simulink model "sampleModel137"  (R2021b)
settings: Solver=VariableStepAuto  StartTime=0.0  StopTime=10.0  RelTol=1e-3
undefined symbols (not defined in the file or in its folder): Newton, Raphson
libraries: simulink x11, slpidlib x2
settings Model: Creator=user  LastModifiedBy=user

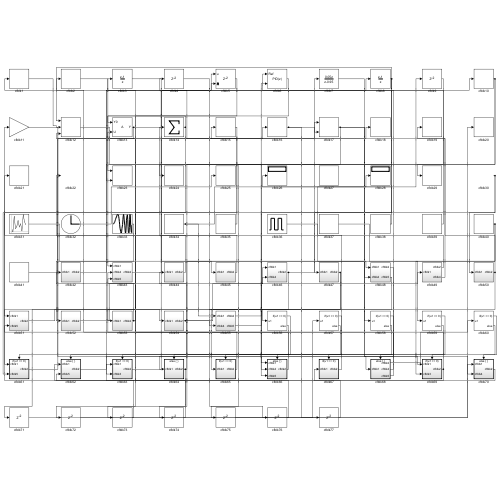
[thumbnail: Simulink's stored preview of the top-level diagram]
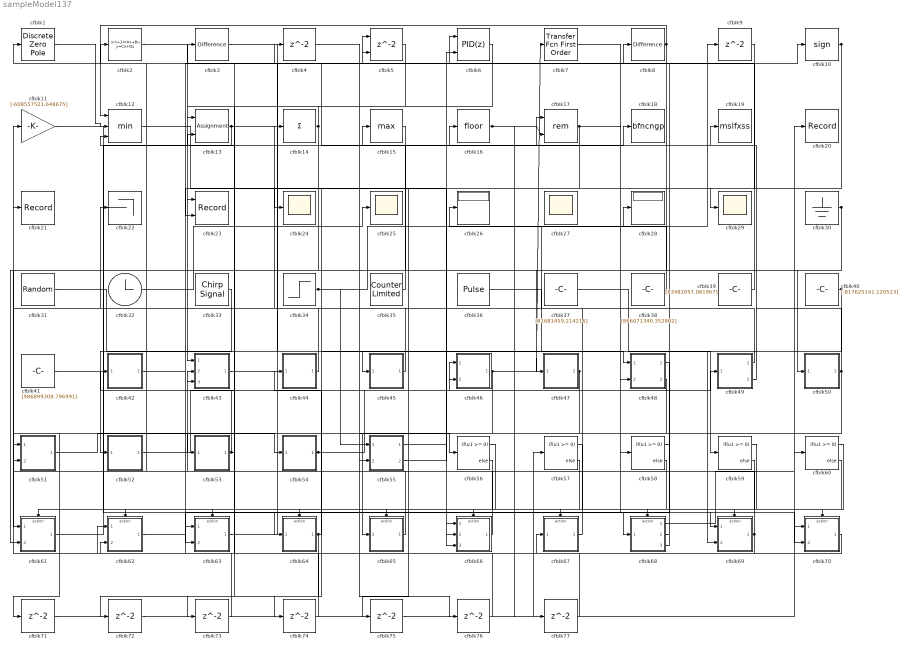
== system sampleModel137 ==
  cfblk1 : DiscreteZeroPole  Poles=[0 0.5]  Gain=1
  cfblk10 : Signum
  cfblk11 : Gain  Gain=[-608557521.648675]
  cfblk12 : MinMax  Inputs=3
  cfblk13 : Assignment  DiagnosticForDimensions=Warning  IndexOptions=Index vector (dialog)  Indices=1  OutputSizes=1
  cfblk14 : Sum  Inputs=+
  cfblk15 : MinMax  Function=max
  cfblk16 : Rounding
  cfblk17 : Math  Operator=rem  SaturateOnIntegerOverflow=on
  cfblk18 : ToWorkspace  VariableName=bfncngp  SaveFormat=Timeseries  SampleTime=-1
  cfblk19 : ToWorkspace  VariableName=mslfxss  SaveFormat=Timeseries  SampleTime=-1
  cfblk2 : DiscreteStateSpace
  cfblk20 : Record  FileSettingsInternal="{\"entries\":[{\"content\":{\"excelSettings\":{\"content\":{},\"type\":\"Streamout.ExcelSettings\"}},\"type\":\"Streamout.FileSettingStorage\",\"uuid\":\"78cab240-d707-46c0-bab2-71765f668cae\"}],\"packageUris\":[\"http://schema.mathworks.com/mf0/streamout_blocks/R2020a\"],\"version\":\"1.0\"}"  SignalsInternal="{\"entries\":[{\"content\":{\"signals\":[{\"content\":{\"blockPath\":[\"sampleModel137/cfblk20\"],\"channel\":[],\"dimensions\":[1],\"domain\":\"sampleModel137/cfblk20\",\"lineColor\":\"#77ac30\",\"plots\":[1],\"port\":1,\"sid\":[\"\"],\"signalID\":4817,\"signalName\":\"cfblk68:1\"},\"type\":\"RecordBlkView.Signal\",\"uuid\":\"5ba74064-0a93-45ca-96c5-9e64b5215f86\"}]},\"type\":\"RecordBlkView.InputSignals\",\"uuid\":\"459eb6df-0716-4f70-a343-e867666ea349\"}],\"packageUris\":[\"http://schema.mathworks.com/mf0/streamout_blocks/R2020a\"],\"version\":\"1.0\"}"  VisualizationBindings="{\"sparklinesplugin\":{\"info\":[{\"bindingParametersList\":[],\"subplotID\":1}]}}"
  cfblk21 : Record  FileSettingsInternal="{\"entries\":[{\"content\":{\"excelSettings\":{\"content\":{},\"type\":\"Streamout.ExcelSettings\"}},\"type\":\"Streamout.FileSettingStorage\",\"uuid\":\"bc3cb0e1-2b9a-4902-8bb5-5abf4e2b3de7\"}],\"packageUris\":[\"http://schema.mathworks.com/mf0/streamout_blocks/R2020a\"],\"version\":\"1.0\"}"  SignalsInternal="{\"entries\":[{\"content\":{\"signals\":[{\"content\":{\"blockPath\":[\"sampleModel137/cfblk21\"],\"channel\":[],\"dimensions\":[1],\"domain\":\"sampleModel137/cfblk21\",\"lineColor\":\"#4dbeee\",\"plots\":[1],\"port\":1,\"sid\":[\"\"],\"signalID\":4821,\"signalName\":\"cfblk49:1\"},\"type\":\"RecordBlkView.Signal\",\"uuid\":\"d4e94c7a-f449-4d3a-8495-2eef223feb6d\"}]},\"type\":\"RecordBlkView.InputSignals\",\"uuid\":\"f1cf74e8-d586-40d0-87c1-09232b5e8770\"}],\"packageUris\":[\"http://schema.mathworks.com/mf0/streamout_blocks/R2020a\"],\"version\":\"1.0\"}"  VisualizationBindings="{\"sparklinesplugin\":{\"info\":[{\"bindingParametersList\":[],\"subplotID\":1}]}}"
  cfblk22 : Terminator
  cfblk23 : Record  FileSettingsInternal="{\"entries\":[{\"content\":{\"excelSettings\":{\"content\":{},\"type\":\"Streamout.ExcelSettings\"}},\"type\":\"Streamout.FileSettingStorage\",\"uuid\":\"2b119019-7ec8-40aa-a939-0d8a92bc28e8\"}],\"packageUris\":[\"http://schema.mathworks.com/mf0/streamout_blocks/R2020a\"],\"version\":\"1.0\"}"  Layout=[1 1]  SignalsInternal="{\"entries\":[{\"content\":{\"signals\":[{\"content\":{\"blockPath\":[\"sampleModel137/cfblk23\"],\"channel\":[],\"dimensions\":[1],\"domain\":\"sampleModel137/cfblk23\",\"lineColor\":\"#a2142f\",\"plots\":[1],\"port\":1,\"sid\":[\"\"],\"signalID\":4825,\"signalName\":\"cfblk2\"},\"type\":\"RecordBlkView.Signal\",\"uuid\":\"4b9917a8-76f8-4205-8d4f-0c51dee1f9f1\"},{\"content\":{\"blockPath\":[\"sampleModel137/cfblk23\"],\"channel\":[],\"dimensions\":[1],\"domain\":\"sampleModel137/cfblk23\",\"lineColor\":\"#139fff\",\"plots\":[1],\"port\":2,\"sid\":[\"\"],\"signalID\":4829,\"signalName\":\"cfblk8\"},\"type\":\"RecordBlkView.Signal\",\"uuid\":\"6d67ff03-11df-4e94-8c93-0e4ad8945509\"}]},\"type\":\"RecordBlkView.InputSignals\",\"uuid\":\"666818d9-2857-43ed-83f7-2c87851fb6a0\"}],\"packageUris\":[\"http://schema.mathworks.com/mf0/streamout_blocks/R2020a\"],\"version\":\"1.0\"}"  VisualizationBindings="{\"xyplotplugin\":{\"info\":[{\"series\":[{\"bindingParametersList\":[{\"parameter\":\"X-Axis\",\"signalID\":4825,\"signalName\":\"cfblk2\"},{\"parameter\":\"Y-Axis\",\"signalID\":4829,\"signalName\":\"cfblk8\"}],\"seriesID\":38646}],\"subplotID\":1}]}}"  CompatibilityTag=XY
  cfblk{24..25,27,29} (4 alike) : Scope
      cfblk27 settings: Floating=on
  cfblk26 : Display
  cfblk28 : Display
  cfblk3 : simulink/Discrete/Difference  ICPrevInput=0.0  OutMin=[]  OutMax=[]  OutDataTypeStr=Inherit: Inherit via back propagation  OutDataType=fixdt(1, 16)  OutScaling=2^-10  DoSatur=off
  cfblk30 : Ground
  cfblk31 : UniformRandomNumber  Minimum=[-3748405739.129770]  Maximum=[821587507.931127]  Seed=[41408692.000000]  SampleTime=0.1
  cfblk32 : Clock
  cfblk33 : simulink/Sources/Chirp Signal  f1=[-767972727.541199]  T=[-712387255.686260]  f2=[-738872032.789923]
  cfblk34 : Step  Time=[44.000000]  Before=[-628794468.071128]  After=[-424292233.508765]  SampleTime=0
  cfblk35 : simulink/Sources/Counter Limited  uplimit=[466.000000]  tsamp=-1
  cfblk36 : DiscretePulseGenerator  PulseType=Time based  Amplitude=[628298384.607478]  Period=[32439850.198564]  PulseWidth=5  PhaseDelay=[8.000000]
  cfblk37 : Constant  Value=[81681459.214216]  SampleTime=1
  cfblk38 : Constant  Value=[866071340.352802]  SampleTime=1
  cfblk39 : Constant  Value=[83482057.081967]  SampleTime=1
  cfblk{4,9,71..77} (9 alike) : Delay  SampleTime=1
  cfblk40 : Constant  Value=[-817625141.120523]  SampleTime=1
  cfblk41 : Constant  Value=[986899308.796991]  SampleTime=1
  cfblk42 : Subsystem
  cfblk43 : Subsystem
  cfblk44 : Subsystem
  cfblk45 : Subsystem
  cfblk46 : Subsystem
  cfblk47 : Subsystem
  cfblk48 : Subsystem
  cfblk49 : Subsystem
  cfblk5 : Delay  ShowEnablePort=on  SampleTime=1
      settings: InputPortMap=u0,e6
  cfblk50 : Subsystem
  cfblk51 : Subsystem
  cfblk52 : Subsystem
  cfblk53 : Subsystem
  cfblk54 : Subsystem
  cfblk55 : Subsystem
  cfblk{56..60} (5 alike) : If  IfExpression=u1 >= 0  SampleTime=1
  cfblk6 : slpidlib/PID Controller (2DOF)  Controller=PID  Form=Parallel  TimeDomain=Discrete-time  UseExternalTs=off  SampleTime=1  IntegratorMethod=Forward Euler  FilterMethod=Forward Euler  ControllerParametersSource=internal  P=1  I=1  D=0  UseFilter=on  N=100  b=1  c=1  TunerSelectOption=Transfer Function Based (PID Tuner App)  InitialConditionSource=internal  InitialConditionForIntegrator=0  InitialConditionForFilter=0  DifferentiatorICPrevScaledInput=0  ExternalReset=none  TrackingMode=off  Kt=1  LimitOutput=off  SatLimitsSource=internal  UpperSaturationLimit=inf  LowerSaturationLimit=-inf  LinearizeAsGain=off  AntiWindupMode=none  Kb=1  POutMin=[]  POutMax=[]  IOutMin=[]  IOutMax=[]  DOutMin=[]  DOutMax=[]  NOutMin=[]  NOutMax=[]  bOutMin=[]  bOutMax=[]  cOutMin=[]  cOutMax=[]  SumOutMin=[]  SumOutMax=[]  SaturationOutMin=[]  SaturationOutMax=[]  PParamMin=[]  PParamMax=[]  IParamMin=[]  IParamMax=[]  DParamMin=[]  DParamMax=[]  NParamMin=[]  NParamMax=[]  bParamMin=[]  bParamMax=[]  cParamMin=[]  cParamMax=[]  KbParamMin=[]  KbParamMax=[]  KtParamMin=[]  KtParamMax=[]  KbOutMin=[]  KbOutMax=[]  KtOutMin=[]  KtOutMax=[]  IntegratorOutMin=[]  IntegratorOutMax=[]  FilterOutMin=[]  FilterOutMax=[]  SumI1OutMin=[]  SumI1OutMax=[]  SumI2OutMin=[]  SumI2OutMax=[]  SumI3OutMin=[]  SumI3OutMax=[]  SumI4OutMin=[]  SumI4OutMax=[]  SumDOutMin=[]  SumDOutMax=[]  Sum1OutMin=[]  Sum1OutMax=[]  Sum2OutMin=[]  Sum2OutMax=[]  Sum3OutMin=[]  Sum3OutMax=[]  DifferentiatorOutMin=[]  DifferentiatorOutMax=[]  FilterDiffOutCoefMin=[]  FilterDiffOutCoefMax=[]  ReciprocalOutMin=[]  ReciprocalOutMax=[]  SumDenOutMin=[]  SumDenOutMax=[]  SumNumOutMin=[]  SumNumOutMax=[]  DivideOutMin=[]  DivideOutMax=[]  UdiffTsProdOutMin=[]  UdiffTsProdOutMax=[]  NTsProdOutMin=[]  NTsProdOutMax=[]  UintegralTsProdOutMin=[]  UintegralTsProdOutMax=[]  UngainTsProdOutMin=[]  UngainTsProdOutMax=[]  IntegratorContinuousStateAttributes=''  IntegratorStateMustResolveToSignalObject=off  IntegratorRTWStateStorageClass=Auto  FilterContinuousStateAttributes=''  FilterStateMustResolveToSignalObject=off  FilterRTWStateStorageClass=Auto  ParallelPVariant=InternalParameters  IdealPVariant=Disabled  IVariant=InternalParameters  DVariant=InternalParameters  bVariant=InternalParameters  cVariant=InternalParameters  IntegratorVariant=Discrete  SatVariant=Disabled  AWVariant=Passthrough  PCopyVariant=Disabled  TRVariant=Disabled  FdbkBlocksVariant=Forward  IdealPFdbkVariant=Disabled  SatFdbkVariant=Disabled  DerivativeFilterVariant=ForwardEulerFilter  NVariant=InternalParameters  NCopyVariant=Disabled  FilterICVariant=InternalICsFilter  IntegratorICVariant=InternalICs  ExternalResetVariant=Disabled  TRSumVariant=Passthrough  SumFdbkVariant=Disabled  SumVariant=Sum_PID  TsampFilterVariant=InternalTs  TsampNgainVariant=Passthrough  TsampIntegralVariant=Passthrough  ExternalSaturationOutDataTypeStr=Inherit: Same as second input
      settings: SourceProductBaseCode=SL
  cfblk61 : Subsystem  TreatAsAtomicUnit=on
  cfblk62 : Subsystem  TreatAsAtomicUnit=on
  cfblk63 : Subsystem  TreatAsAtomicUnit=on
  cfblk64 : Subsystem  TreatAsAtomicUnit=on
  cfblk65 : Subsystem  TreatAsAtomicUnit=on
  cfblk66 : Subsystem  TreatAsAtomicUnit=on
  cfblk67 : Subsystem  TreatAsAtomicUnit=on
  cfblk68 : Subsystem  TreatAsAtomicUnit=on
  cfblk69 : Subsystem  TreatAsAtomicUnit=on
  cfblk7 : simulink/Discrete/Transfer Fcn First Order  PoleZ=0.95  ICPrevOutput=0.0  DoSatur=off
  cfblk70 : Subsystem  TreatAsAtomicUnit=on
  cfblk8 : simulink/Discrete/Difference  ICPrevInput=0.0  OutMin=[]  OutMax=[]  OutDataTypeStr=Inherit: Inherit via back propagation  OutDataType=fixdt(1, 16)  OutScaling=2^-10  DoSatur=off
  wires:
  cfblk37/1 -> cfblk59/1
  cfblk9/1 -> cfblk29/1
  cfblk63/1(cfblk2) -> cfblk8/1
  cfblk67/1(cfblk2) -> cfblk28/1
  cfblk46/1(cfblk2) -> cfblk7/1, cfblk71/1
  cfblk70/1(cfblk2) -> cfblk11/1
  cfblk61/1(cfblk2) -> cfblk16/1
  cfblk64/1(cfblk2) -> cfblk44/1(cfblk1), cfblk72/1
  cfblk10/1 -> cfblk74/1, cfblk75/1
  cfblk11/1 -> cfblk68/1(cfblk1)
  cfblk5/1 -> cfblk43/1(cfblk1)
  cfblk13/1 -> cfblk5/1, cfblk12/3
  cfblk52/1(cfblk2) -> cfblk46/1(cfblk1)
  cfblk31/1 -> cfblk45/1(cfblk1)
  cfblk41/1 -> cfblk17/1
  cfblk42/1(cfblk2) -> cfblk5/2
  cfblk8/1 -> cfblk12/1, cfblk61/2(cfblk5), cfblk23/2, cfblk66/3(cfblk5)
  cfblk1/1 -> cfblk12/2
  cfblk62/1(cfblk2) -> cfblk10/1
  cfblk54/1(cfblk2) -> cfblk46/2(cfblk4), cfblk76/1
  cfblk53/1(cfblk2) -> cfblk2/1, cfblk13/2
  cfblk49/1(cfblk2) -> cfblk21/1
  cfblk2/1 -> cfblk23/1
  cfblk69/1(cfblk2) -> cfblk67/1(cfblk1), cfblk43/3(cfblk5)
  cfblk33/1 -> cfblk52/1(cfblk1)
  cfblk15/1 -> cfblk61/1(cfblk1)
  cfblk7/1 -> cfblk58/1
  cfblk43/1(cfblk2) -> cfblk18/1
  cfblk66/1(cfblk2) -> cfblk42/1(cfblk1)
  cfblk30/1 -> cfblk47/1(cfblk1), cfblk50/1(cfblk1)
  cfblk3/1 -> cfblk48/1(cfblk1)
  cfblk47/1(cfblk2) -> cfblk51/1(cfblk1), cfblk66/2(cfblk4)
  cfblk32/1 -> cfblk25/1
  cfblk65/1(cfblk2) -> cfblk43/2(cfblk4)
  cfblk39/1 -> cfblk6/1
  cfblk55/1(cfblk2) -> cfblk6/2
  cfblk12/1 -> cfblk66/1(cfblk1)
  cfblk49/2(cfblk4) -> cfblk15/1
  cfblk44/1(cfblk2) -> cfblk14/1
  cfblk34/1 -> cfblk9/1, cfblk55/1(cfblk1)
  cfblk14/1 -> cfblk13/1, cfblk73/1
  cfblk35/1 -> cfblk4/1
  cfblk51/1(cfblk2) -> cfblk54/1(cfblk1)
  cfblk68/1(cfblk2) -> cfblk20/1
  cfblk16/1 -> cfblk17/2, cfblk77/1
  cfblk36/1 -> cfblk48/2(cfblk4)
  cfblk4/1 -> cfblk56/1
  cfblk6/1 -> cfblk53/1(cfblk1)
  cfblk45/1(cfblk2) -> cfblk22/1
  cfblk40/1 -> cfblk64/1(cfblk1), cfblk69/2(cfblk3)
  cfblk50/1(cfblk2) -> cfblk19/1, cfblk55/2(cfblk4)
  cfblk55/2(cfblk5) -> cfblk49/1(cfblk1)
  cfblk68/2(cfblk4) -> cfblk51/2(cfblk5)
  cfblk68/3(cfblk5) -> cfblk1/1
  cfblk38/1 -> cfblk26/1
  cfblk48/1(cfblk2) -> cfblk63/2(cfblk3)
  cfblk17/1 -> cfblk69/1(cfblk1), cfblk24/1, cfblk70/2(cfblk4)
  cfblk48/2(cfblk5) -> cfblk65/1(cfblk1)
  cfblk56/1 -> cfblk61/Action
  cfblk56/2 -> cfblk62/Action
  cfblk57/1 -> cfblk63/Action
  cfblk57/2 -> cfblk64/Action
  cfblk58/1 -> cfblk65/Action
  cfblk58/2 -> cfblk66/Action
  cfblk59/1 -> cfblk67/Action
  cfblk59/2 -> cfblk68/Action
  cfblk60/1 -> cfblk69/Action
  cfblk60/2 -> cfblk70/Action
  cfblk71/1 -> cfblk57/1
  cfblk72/1 -> cfblk60/1
  cfblk73/1 -> cfblk62/2(cfblk5)
  cfblk74/1 -> cfblk63/1(cfblk1)
  cfblk75/1 -> cfblk70/1(cfblk1)
  cfblk76/1 -> cfblk62/1(cfblk1)
  cfblk77/1 -> cfblk3/1

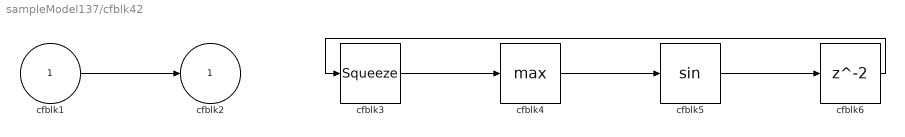
== system sampleModel137/cfblk42 ==
  cfblk1 : Inport
  cfblk3 : Squeeze
  cfblk4 : MinMax  Function=max
  cfblk5 : Trigonometry
  cfblk6 : Delay  SampleTime=1
  cfblk2 : Outport
  wires:
  cfblk3/1 -> cfblk4/1
  cfblk4/1 -> cfblk5/1
  cfblk1/1 -> cfblk2/1
  cfblk5/1 -> cfblk6/1
  cfblk6/1 -> cfblk3/1

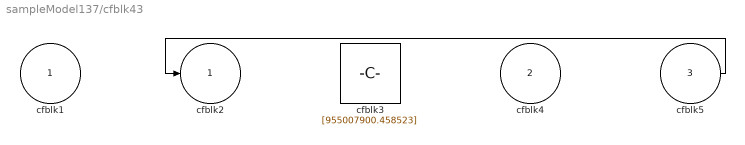
== system sampleModel137/cfblk43 ==
  cfblk1 : Inport
  cfblk4 : Inport  Port=2
  cfblk5 : Inport  Port=3
  cfblk3 : Constant  Value=[955007900.458523]  SampleTime=1
  cfblk2 : Outport
  wires:
  cfblk5/1 -> cfblk2/1

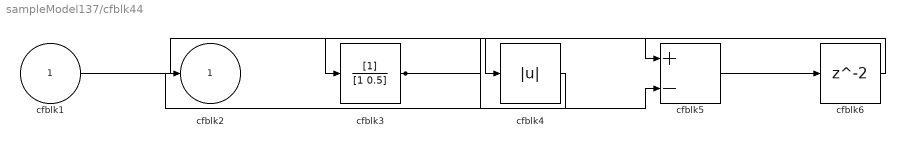
== system sampleModel137/cfblk44 ==
  cfblk1 : Inport
  cfblk3 : DiscreteFilter  SampleTime=1
  cfblk4 : Abs
  cfblk5 : Sum  Inputs=+-
  cfblk6 : Delay  SampleTime=1
  cfblk2 : Outport
  wires:
  cfblk1/1 -> cfblk4/1
  cfblk4/1 -> cfblk2/1
  cfblk3/1 -> cfblk5/1, cfblk5/2
  cfblk5/1 -> cfblk6/1
  cfblk6/1 -> cfblk3/1

== system sampleModel137/cfblk45 ==
  cfblk1 : Inport
  cfblk3 : Bias  Bias=[-716241276.634406]
  cfblk4 : Product
  cfblk2 : Outport
  wires:
  cfblk1/1 -> cfblk3/1, cfblk4/2
  cfblk3/1 -> cfblk2/1, cfblk4/1

== system sampleModel137/cfblk46 ==
  cfblk1 : Inport
  cfblk4 : Inport  Port=2
  cfblk3 : Product  Inputs=*
  cfblk2 : Outport
  wires:
  cfblk3/1 -> cfblk2/1
  cfblk4/1 -> cfblk3/1

== system sampleModel137/cfblk47 ==
  cfblk1 : Inport
  cfblk3 : Sum  Inputs=+
  cfblk2 : Outport
  wires:
  cfblk1/1 -> cfblk3/1
  cfblk3/1 -> cfblk2/1

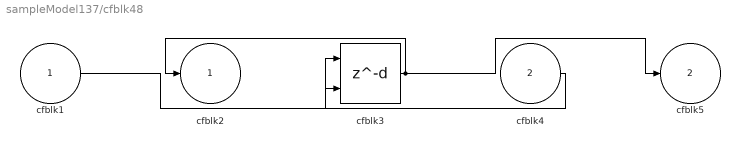
== system sampleModel137/cfblk48 ==
  cfblk1 : Inport
  cfblk4 : Inport  Port=2
  cfblk3 : Delay  DelayLengthSource=Input port  SampleTime=1
      settings: InputPortMap=u0,p1
  cfblk2 : Outport
  cfblk5 : Outport  Port=2
  wires:
  cfblk3/1 -> cfblk2/1, cfblk5/1
  cfblk4/1 -> cfblk3/1
  cfblk1/1 -> cfblk3/2

== system sampleModel137/cfblk49 ==
  cfblk1 : Inport
  cfblk3 : Constant  Value=[-479346277.311574]  SampleTime=1
  cfblk2 : Outport
  cfblk4 : Outport  Port=2
  wires:
  cfblk1/1 -> cfblk4/1
  cfblk3/1 -> cfblk2/1

== system sampleModel137/cfblk50 ==
  cfblk1 : Inport
  cfblk3 : simulink/Discrete/Transfer Fcn Lead or Lag  PoleZ=0.95  ZeroZ=0.75  ICPrevOutput=0.0  ICPrevInput=0.0  DoSatur=off
      settings: SourceProductBaseCode=SL
  cfblk4 : Constant  Value=[195739199.430288]  SampleTime=1
  cfblk2 : Outport
  wires:
  cfblk1/1 -> cfblk2/1
  cfblk4/1 -> cfblk3/1

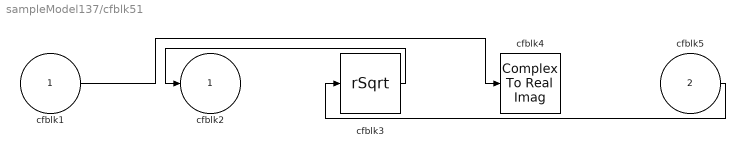
== system sampleModel137/cfblk51 ==
  cfblk1 : Inport
  cfblk5 : Inport  Port=2
  cfblk3 : Sqrt  Operator=rSqrt  AlgorithmType=Newton-Raphson  SaturateOnIntegerOverflow=on
  cfblk4 : ComplexToRealImag
  cfblk2 : Outport
  wires:
  cfblk3/1 -> cfblk2/1
  cfblk5/1 -> cfblk3/1
  cfblk1/1 -> cfblk4/1

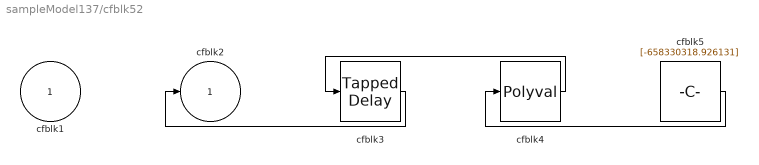
== system sampleModel137/cfblk52 ==
  cfblk1 : Inport
  cfblk3 : simulink/Discrete/Tapped Delay  vinit=0.0  samptime=-1  NumDelays=1  DelayOrder=Oldest  includeCurrent=off
  cfblk4 : Polyval  Coefs=[ +2.081618890e-019, -1.441693666e-014, +4.719686976e-010, -8.536869453e-006, +1.621573104e-001, -8.087801117e+001 ]
  cfblk5 : Constant  Value=[-658330318.926131]  SampleTime=1
  cfblk2 : Outport
  wires:
  cfblk4/1 -> cfblk3/1
  cfblk5/1 -> cfblk4/1
  cfblk3/1 -> cfblk2/1

== system sampleModel137/cfblk53 ==
  cfblk1 : Inport
  cfblk3 : ComplexToMagnitudeAngle
  cfblk2 : Outport
  wires:
  cfblk1/1 -> cfblk2/1, cfblk3/1

== system sampleModel137/cfblk54 ==
  cfblk1 : Inport
  cfblk3 : UnitDelay  HasFrameUpgradeWarning=on
  cfblk4 : simulink/Math Operations/Slider Gain  gain=1  low=0  high=2
  cfblk2 : Outport
  wires:
  cfblk1/1 -> cfblk3/1
  cfblk3/1 -> cfblk4/1
  cfblk4/1 -> cfblk2/1

== system sampleModel137/cfblk55 ==
  cfblk1 : Inport
  cfblk4 : Inport  Port=2
  cfblk3 : Squeeze
  cfblk2 : Outport
  cfblk5 : Outport  Port=2
  wires:
  cfblk3/1 -> cfblk2/1
  cfblk1/1 -> cfblk3/1
  cfblk4/1 -> cfblk5/1

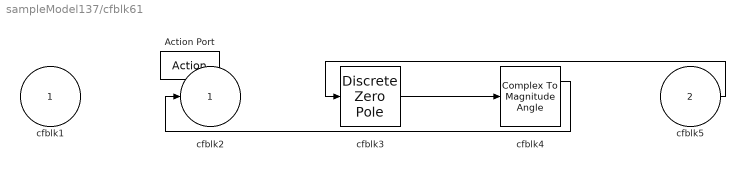
== system sampleModel137/cfblk61 ==
  cfblk1 : Inport
  cfblk5 : Inport  Port=2
  Action Port : ActionPort  ActionPortLabel=if(u1 >= 0)
  cfblk3 : DiscreteZeroPole  Poles=[0 0.5]  Gain=1  SampleTime=-1
  cfblk4 : ComplexToMagnitudeAngle
  cfblk2 : Outport
  wires:
  cfblk5/1 -> cfblk3/1
  cfblk4/1 -> cfblk2/1
  cfblk3/1 -> cfblk4/1

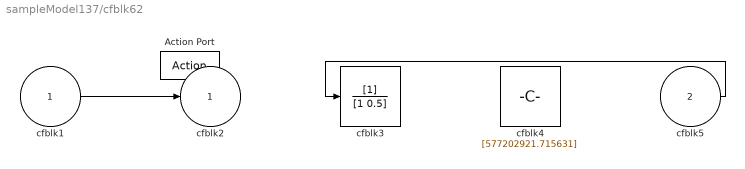
== system sampleModel137/cfblk62 ==
  cfblk1 : Inport
  cfblk5 : Inport  Port=2
  Action Port : ActionPort  ActionPortLabel=else
  cfblk3 : DiscreteFilter
  cfblk4 : Constant  Value=[577202921.715631]  SampleTime=1
  cfblk2 : Outport
  wires:
  cfblk1/1 -> cfblk2/1
  cfblk5/1 -> cfblk3/1

== system sampleModel137/cfblk63 ==
  cfblk1 : Inport
  cfblk3 : Inport  Port=2
  Action Port : ActionPort  ActionPortLabel=if(u1 >= 0)
  cfblk2 : Outport
  wires:
  cfblk3/1 -> cfblk2/1

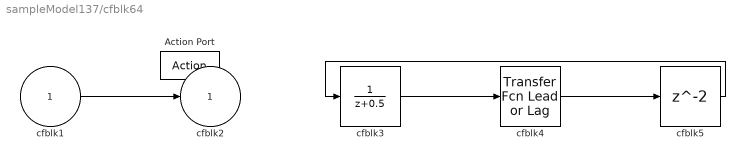
== system sampleModel137/cfblk64 ==
  cfblk1 : Inport
  Action Port : ActionPort  ActionPortLabel=else
  cfblk3 : DiscreteTransferFcn
  cfblk4 : simulink/Discrete/Transfer Fcn Lead or Lag  PoleZ=0.95  ZeroZ=0.75  ICPrevOutput=0.0  ICPrevInput=0.0  DoSatur=off
      settings: SourceProductBaseCode=SL
  cfblk5 : Delay
  cfblk2 : Outport
  wires:
  cfblk1/1 -> cfblk2/1
  cfblk3/1 -> cfblk4/1
  cfblk4/1 -> cfblk5/1
  cfblk5/1 -> cfblk3/1

== system sampleModel137/cfblk65 ==
  cfblk1 : Inport
  Action Port : ActionPort  ActionPortLabel=if(u1 >= 0)
  cfblk3 : simulink/Discrete/Transfer Fcn Real Zero  ZeroZ=0.75  ICPrevInput=0.0  DoSatur=off
      settings: SourceProductBaseCode=SL
  cfblk4 : Constant  Value=[632609571.556403]  SampleTime=1
  cfblk2 : Outport
  wires:
  cfblk4/1 -> cfblk3/1
  cfblk3/1 -> cfblk2/1

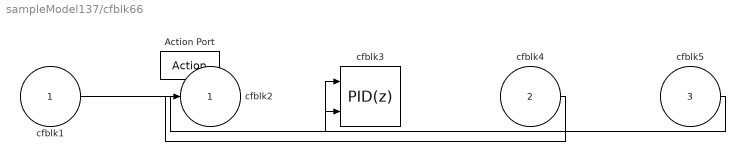
== system sampleModel137/cfblk66 ==
  cfblk1 : Inport
  cfblk4 : Inport  Port=2
  cfblk5 : Inport  Port=3
  Action Port : ActionPort  ActionPortLabel=else
  cfblk3 : slpidlib/PID Controller (2DOF)  Controller=PID  Form=Parallel  TimeDomain=Discrete-time  UseExternalTs=off  SampleTime=-1  IntegratorMethod=Forward Euler  FilterMethod=Forward Euler  ControllerParametersSource=internal  P=1  I=1  D=0  UseFilter=on  N=100  b=1  c=1  TunerSelectOption=Transfer Function Based (PID Tuner App)  InitialConditionSource=internal  InitialConditionForIntegrator=0  InitialConditionForFilter=0  DifferentiatorICPrevScaledInput=0  ExternalReset=none  TrackingMode=off  Kt=1  LimitOutput=off  SatLimitsSource=internal  UpperSaturationLimit=inf  LowerSaturationLimit=-inf  LinearizeAsGain=off  AntiWindupMode=none  Kb=1  POutMin=[]  POutMax=[]  IOutMin=[]  IOutMax=[]  DOutMin=[]  DOutMax=[]  NOutMin=[]  NOutMax=[]  bOutMin=[]  bOutMax=[]  cOutMin=[]  cOutMax=[]  SumOutMin=[]  SumOutMax=[]  SaturationOutMin=[]  SaturationOutMax=[]  PParamMin=[]  PParamMax=[]  IParamMin=[]  IParamMax=[]  DParamMin=[]  DParamMax=[]  NParamMin=[]  NParamMax=[]  bParamMin=[]  bParamMax=[]  cParamMin=[]  cParamMax=[]  KbParamMin=[]  KbParamMax=[]  KtParamMin=[]  KtParamMax=[]  KbOutMin=[]  KbOutMax=[]  KtOutMin=[]  KtOutMax=[]  IntegratorOutMin=[]  IntegratorOutMax=[]  FilterOutMin=[]  FilterOutMax=[]  SumI1OutMin=[]  SumI1OutMax=[]  SumI2OutMin=[]  SumI2OutMax=[]  SumI3OutMin=[]  SumI3OutMax=[]  SumI4OutMin=[]  SumI4OutMax=[]  SumDOutMin=[]  SumDOutMax=[]  Sum1OutMin=[]  Sum1OutMax=[]  Sum2OutMin=[]  Sum2OutMax=[]  Sum3OutMin=[]  Sum3OutMax=[]  DifferentiatorOutMin=[]  DifferentiatorOutMax=[]  FilterDiffOutCoefMin=[]  FilterDiffOutCoefMax=[]  ReciprocalOutMin=[]  ReciprocalOutMax=[]  SumDenOutMin=[]  SumDenOutMax=[]  SumNumOutMin=[]  SumNumOutMax=[]  DivideOutMin=[]  DivideOutMax=[]  UdiffTsProdOutMin=[]  UdiffTsProdOutMax=[]  NTsProdOutMin=[]  NTsProdOutMax=[]  UintegralTsProdOutMin=[]  UintegralTsProdOutMax=[]  UngainTsProdOutMin=[]  UngainTsProdOutMax=[]  IntegratorContinuousStateAttributes=''  IntegratorStateMustResolveToSignalObject=off  IntegratorRTWStateStorageClass=Auto  FilterContinuousStateAttributes=''  FilterStateMustResolveToSignalObject=off  FilterRTWStateStorageClass=Auto  ParallelPVariant=InternalParameters  IdealPVariant=Disabled  IVariant=InternalParameters  DVariant=InternalParameters  bVariant=InternalParameters  cVariant=InternalParameters  IntegratorVariant=Discrete  SatVariant=Disabled  AWVariant=Passthrough  PCopyVariant=Disabled  TRVariant=Disabled  FdbkBlocksVariant=Forward  IdealPFdbkVariant=Disabled  SatFdbkVariant=Disabled  DerivativeFilterVariant=ForwardEulerFilter  NVariant=InternalParameters  NCopyVariant=Disabled  FilterICVariant=InternalICsFilter  IntegratorICVariant=InternalICs  ExternalResetVariant=Disabled  TRSumVariant=Passthrough  SumFdbkVariant=Disabled  SumVariant=Sum_PID  TsampFilterVariant=InternalTs  TsampNgainVariant=Passthrough  TsampIntegralVariant=Passthrough  ExternalSaturationOutDataTypeStr=Inherit: Same as second input
      settings: SourceProductBaseCode=SL
  cfblk2 : Outport
  wires:
  cfblk1/1 -> cfblk3/1
  cfblk4/1 -> cfblk2/1
  cfblk5/1 -> cfblk3/2

== system sampleModel137/cfblk67 ==
  cfblk1 : Inport
  Action Port : ActionPort  ActionPortLabel=if(u1 >= 0)
  cfblk3 : Delay  DelayLengthSource=Input port
      settings: InputPortMap=u0,p1
  cfblk2 : Outport
  wires:
  cfblk1/1 -> cfblk2/1, cfblk3/1, cfblk3/2

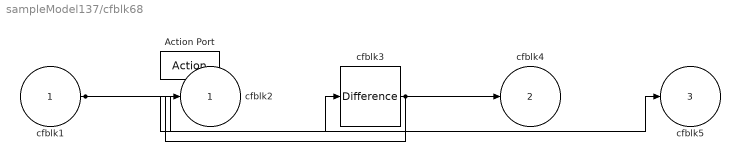
== system sampleModel137/cfblk68 ==
  cfblk1 : Inport
  Action Port : ActionPort  ActionPortLabel=else
  cfblk3 : simulink/Discrete/Difference  ICPrevInput=0.0  OutMin=[]  OutMax=[]  OutDataTypeStr=Inherit: Inherit via back propagation  OutDataType=fixdt(1, 16)  OutScaling=2^-10  DoSatur=off
  cfblk2 : Outport
  cfblk4 : Outport  Port=2
  cfblk5 : Outport  Port=3
  wires:
  cfblk1/1 -> cfblk3/1, cfblk5/1
  cfblk3/1 -> cfblk2/1, cfblk4/1

== system sampleModel137/cfblk69 ==
  cfblk1 : Inport
  cfblk3 : Inport  Port=2
  Action Port : ActionPort  ActionPortLabel=if(u1 >= 0)
  cfblk2 : Outport
  wires:
  cfblk1/1 -> cfblk2/1

== system sampleModel137/cfblk70 ==
  cfblk1 : Inport
  cfblk4 : Inport  Port=2
  Action Port : ActionPort  ActionPortLabel=else
  cfblk3 : Delay  ShowEnablePort=on
      settings: InputPortMap=u0,e6
  cfblk2 : Outport
  wires:
  cfblk1/1 -> cfblk2/1
  cfblk4/1 -> cfblk3/1, cfblk3/2
